simulink model "Control_model_matching_no_lineal"  (R2023a)
settings: Solver=FixedStepAuto  StartTime=0.0  StopTime=70  FixedStep=Ts  RelTol=1e-3
values from neighbouring files (symbols this model uses):
  IMU1_aB = [0.000820278190076 0.00115353439469 0.000894968456123]    [DatosSimulador.mat]
  IMU1_aK = [1.26449540403e-05 4.27040286013e-05 5.33261409146e-05]    [DatosSimulador.mat]
  IMU1_aN = [0.00684624677524 0.00597589835525 0.00590605800971]    [DatosSimulador.mat]
  IMU1_gB = [0.000430438056355 0.000168108439539 0.000519584631547]    [DatosSimulador.mat]
  IMU1_gK = [3.54504736606e-05 3.3319713566e-06 4.94506384712e-05]    [DatosSimulador.mat]
  IMU1_gN = [0.0047084921971 0.00506619736552 0.00340488785878]    [DatosSimulador.mat]
  IMU2_aB = [0.00173700635787 0.00079356651986 0.000918277248275]    [DatosSimulador.mat]
  IMU2_aK = [0.000253509817412 2.45614519372e-05 6.68535212753e-05]    [DatosSimulador.mat]
  IMU2_aN = [0.00535466242582 0.00533867441118 0.00558323645964]    [DatosSimulador.mat]
  IMU2_gB = [0.000335599994287 0.000795064377598 0.00045980210416]    [DatosSimulador.mat]
  IMU2_gK = [3.18091115332e-05 5.54514226678e-05 3.22930100083e-05]    [DatosSimulador.mat]
  IMU2_gN = [0.00695891398937 0.00398353487253 0.00368572026491]    [DatosSimulador.mat]
  IMU3_aB = [0.000325683271512 0.000441587151727 0.000601047067903]    [DatosSimulador.mat]
  IMU3_aK = [1.00979314084e-05 2.18555360334e-05 3.5534689232e-05]    [DatosSimulador.mat]
  IMU3_aN = [0.00413628574461 0.00448110466823 0.00368606415577]    [DatosSimulador.mat]
  IMU3_gB = [0.000501559406985 0.000889874761924 0.000218087094254]    [DatosSimulador.mat]
  IMU3_gK = [1.959913061e-05 4.03655103582e-05 4.44406532552e-06]    [DatosSimulador.mat]
  IMU3_gN = [0.00573350535706 0.0096154846251 0.00568739091977]    [DatosSimulador.mat]
  Ts = 0.001    [DatosSimulador.mat]
  TsMot = 0.001    [DatosSimulador.mat]
  TsPos = 0.002    [DatosSimulador.mat]
  TsRef = 0.02    [DatosSimulador.mat]
  TsSenB = 0.001    [DatosSimulador.mat]
  TsSenF = 0.001    [DatosSimulador.mat]
  TsVel = 0.001    [DatosSimulador.mat]
undefined symbols (not defined in the file or in its folder): denG, denM, numG, numM
libraries: mspsensorlib x3, simulink x2
(part 2 of 3)

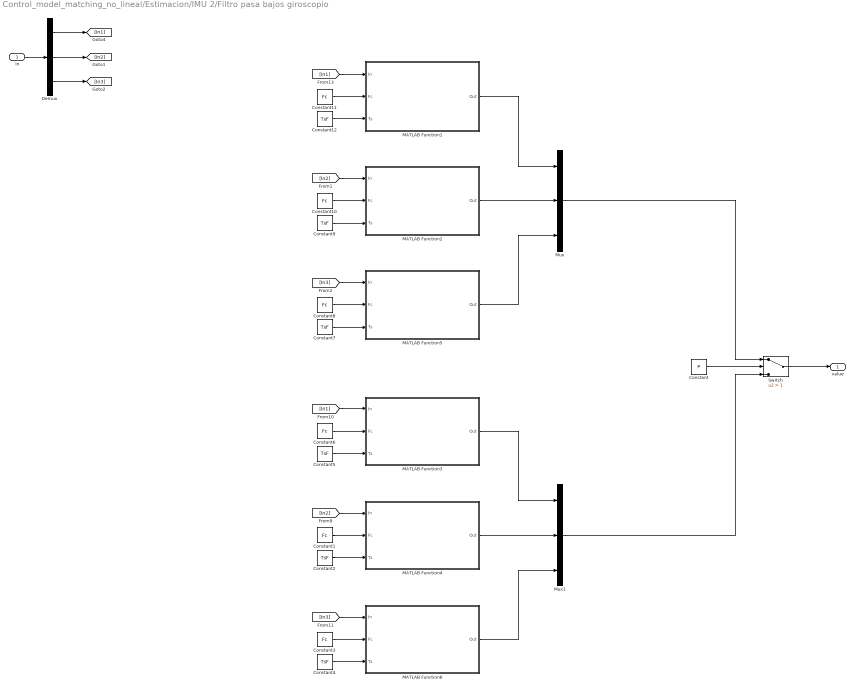
== system Control_model_matching_no_lineal/Estimacion/IMU 2/Filtro pasa bajos giroscopio ==
  In : Inport
  Constant : Constant  Value=P
  Constant{1,3,6,8,10..11} (6 alike) : Constant  Value=Fc
  Constant{2,4..5,7,9,12} (6 alike) : Constant  Value=TsF
  Demux : Demux  Outputs=3
  MATLAB Function1 : MATLAB Function  TreatAsAtomicUnit=on
  MATLAB Function2 : MATLAB Function  TreatAsAtomicUnit=on
  MATLAB Function3 : MATLAB Function  TreatAsAtomicUnit=on
  MATLAB Function4 : MATLAB Function  TreatAsAtomicUnit=on
  MATLAB Function5 : MATLAB Function  TreatAsAtomicUnit=on
  MATLAB Function6 : MATLAB Function  TreatAsAtomicUnit=on
  Mux : Mux  Inputs=3
  Mux1 : Mux  Inputs=3
  Switch : Switch  Criteria=u2 > Threshold  Threshold=1  SaturateOnIntegerOverflow=off  InputSameDT=off
  value : Outport
  wires:
  Constant/1 -> Switch/2
  Switch/1 -> value/1
  [In1] -> MATLAB Function1/1(In)
  MATLAB Function2/1(Out) -> Mux/2
  MATLAB Function1/1(Out) -> Mux/1
  MATLAB Function5/1(Out) -> Mux/3
  Mux/1 -> Switch/1
  In/1 -> Demux/1
  Demux/1 -> [In1]
  Demux/2 -> [In2]
  Demux/3 -> [In3]
  [In2] -> MATLAB Function2/1(In)
  [In3] -> MATLAB Function5/1(In)
  Constant4/1 -> MATLAB Function6/3(Ts)
  Constant3/1 -> MATLAB Function6/2(Fc)
  Constant1/1 -> MATLAB Function4/2(Fc)
  Constant2/1 -> MATLAB Function4/3(Ts)
  [In3] -> MATLAB Function6/1(In)
  [In2] -> MATLAB Function4/1(In)
  [In1] -> MATLAB Function3/1(In)
  MATLAB Function3/1(Out) -> Mux1/1
  MATLAB Function4/1(Out) -> Mux1/2
  MATLAB Function6/1(Out) -> Mux1/3
  Mux1/1 -> Switch/3
  Constant5/1 -> MATLAB Function3/3(Ts)
  Constant6/1 -> MATLAB Function3/2(Fc)
  Constant7/1 -> MATLAB Function5/3(Ts)
  Constant8/1 -> MATLAB Function5/2(Fc)
  Constant10/1 -> MATLAB Function2/2(Fc)
  Constant9/1 -> MATLAB Function2/3(Ts)
  Constant12/1 -> MATLAB Function1/3(Ts)
  Constant11/1 -> MATLAB Function1/2(Fc)

== system Control_model_matching_no_lineal/Estimacion/IMU 2/Sensor IMU ==
  GirT : Inport
  AcelT : Inport  Port=2
  Q : Inport  Port=3
  Constant : Constant  Value=R
  Constant1 : Constant  Value=R
  Gain1 : Gain  Gain=pi/180
  Gain3 : Gain  Gain=180/pi
  Gain4 : Gain  Gain=1/9.81
  IMU : mspsensorlib/IMU  DispRefFrame=NED  Temperature=25  MagneticFieldNED=[ 27.5550, -2.4169, -16.0849 ]  MagneticFieldENU=[ -2.4169, 27.5550, 16.0849 ]  SeedDouble=67  SimulateUsing=Code generation  AccelParamsMeasurementRange=156.9048  AccelParamsResolution=0  AccelParamsConstantBias=[0.0 0.0 0.0]  AccelParamsAxesMisalignment=[0 0 0]  AccelParamsNoiseDensity=aN  AccelParamsBiasInstability=aB  AccelParamsRandomWalk=aK  AccelParamsTemperatureBias=[0 0 0]  AccelParamsTemperatureScaleFactor=[0 0 0]  GyroParamsMeasurementRange=34.9066  GyroParamsResolution=0  GyroParamsConstantBias=[0.0 0.0 0.0]  GyroParamsAxesMisalignment=0  GyroParamsAccelerationBias=[0 0 0]  GyroParamsNoiseDensity=gN  GyroParamsBiasInstability=gB  GyroParamsRandomWalk=gK  GyroParamsTemperatureBias=[0 0 0]  GyroParamsTemperatureScaleFactor=[0 0 0]  MagParamsMeasurementRange=1000  MagParamsResolution=0.1  MagParamsConstantBias=0  MagParamsAxesMisalignment=[0 0 0]  MagParamsNoiseDensity=[0.0424 0.0424 0.0424]  MagParamsBiasInstability=[0 0 0]  MagParamsRandomWalk=[0 0 0]  MagParamsTemperatureBias=[0 0 0]  MagParamsTemperatureScaleFactor=[0 0 0]
  MATLAB Function5 : MATLAB Function  TreatAsAtomicUnit=on  SystemSampleTime=Ts
  Mux : Mux  Inputs=3
  Mux1 : Mux  Inputs=3
  Random Number : RandomNumber  Variance=0.1492^2*1000  SampleTime=Ts
  Random Number3 : RandomNumber  Variance=0.0154^2*1000  SampleTime=Ts
  Sum : Sum  Inputs=|++
  Sum1 : Sum  Inputs=|++
  Switch1 : Switch  Criteria=u2 > Threshold  SaturateOnIntegerOverflow=off  InputSameDT=off
  Switch2 : Switch  Criteria=u2 > Threshold  SaturateOnIntegerOverflow=off  InputSameDT=off
  Transpose1 : Math  Operator=transpose
  Transpose2 : Math  Operator=transpose
  Transpose3 : Math  Operator=transpose
  Zero-Order Hold : ZeroOrderHold  SampleTime=Ts
  Zero-Order Hold1 : ZeroOrderHold  SampleTime=Ts
  Zero-Order Hold2 : ZeroOrderHold  SampleTime=Ts
  AcelB : Outport
  VelB : Outport  Port=2
  wires:
  Zero-Order Hold2/1 -> MATLAB Function5/2(Q), IMU/3
  Zero-Order Hold1/1 -> MATLAB Function5/1(Wb)
  Zero-Order Hold/1 -> Transpose2/1
  Switch1/1 -> IMU/2
  Switch2/1 -> IMU/1
  Gain1/1 -> Sum1/2, Switch1/3
  Sum1/1 -> Switch1/1
  Constant1/1 -> Switch1/2
  Constant/1 -> Switch2/2
  Sum/1 -> Switch2/1
  Random Number3/1 -> Mux1/3, Mux1/2, Mux1/1
  Mux1/1 -> Sum1/1
  Transpose2/1 -> Sum/2, Switch2/3
  Mux/1 -> Sum/1
  Random Number/1 -> Mux/1, Mux/3, Mux/2
  Q/1 -> Zero-Order Hold2/1
  MATLAB Function5/1(Vel) -> Gain1/1
  Transpose3/1 -> Gain3/1
  IMU/1 -> Transpose1/1
  IMU/2 -> Transpose3/1
  GirT/1 -> Zero-Order Hold1/1
  AcelT/1 -> Zero-Order Hold/1
  Transpose1/1 -> Gain4/1
  Gain4/1 -> AcelB/1
  Gain3/1 -> VelB/1

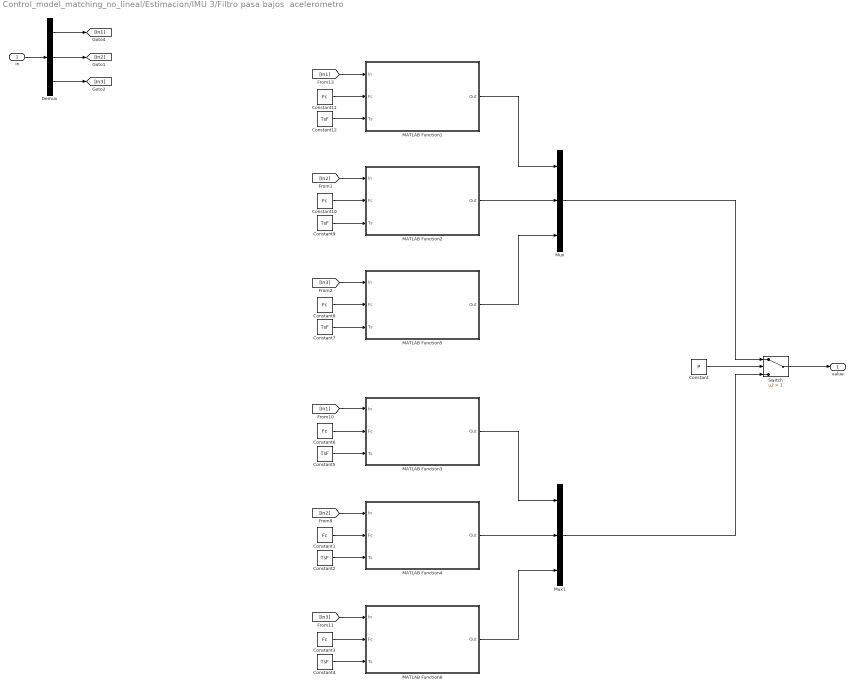
== system Control_model_matching_no_lineal/Estimacion/IMU 3/Filtro pasa bajos  acelerometro ==
  In : Inport
  Constant : Constant  Value=P
  Constant{1,3,6,8,10..11} (6 alike) : Constant  Value=Fc
  Constant{2,4..5,7,9,12} (6 alike) : Constant  Value=TsF
  Demux : Demux  Outputs=3
  MATLAB Function1 : MATLAB Function  TreatAsAtomicUnit=on
  MATLAB Function2 : MATLAB Function  TreatAsAtomicUnit=on
  MATLAB Function3 : MATLAB Function  TreatAsAtomicUnit=on
  MATLAB Function4 : MATLAB Function  TreatAsAtomicUnit=on
  MATLAB Function5 : MATLAB Function  TreatAsAtomicUnit=on
  MATLAB Function6 : MATLAB Function  TreatAsAtomicUnit=on
  Mux : Mux  Inputs=3
  Mux1 : Mux  Inputs=3
  Switch : Switch  Criteria=u2 > Threshold  Threshold=1  SaturateOnIntegerOverflow=off  InputSameDT=off
  value : Outport
  wires:
  Constant/1 -> Switch/2
  Switch/1 -> value/1
  [In1] -> MATLAB Function1/1(In)
  MATLAB Function2/1(Out) -> Mux/2
  MATLAB Function1/1(Out) -> Mux/1
  MATLAB Function5/1(Out) -> Mux/3
  Mux/1 -> Switch/1
  In/1 -> Demux/1
  Demux/1 -> [In1]
  Demux/2 -> [In2]
  Demux/3 -> [In3]
  [In2] -> MATLAB Function2/1(In)
  [In3] -> MATLAB Function5/1(In)
  Constant4/1 -> MATLAB Function6/3(Ts)
  Constant3/1 -> MATLAB Function6/2(Fc)
  Constant1/1 -> MATLAB Function4/2(Fc)
  Constant2/1 -> MATLAB Function4/3(Ts)
  [In3] -> MATLAB Function6/1(In)
  [In2] -> MATLAB Function4/1(In)
  [In1] -> MATLAB Function3/1(In)
  MATLAB Function3/1(Out) -> Mux1/1
  MATLAB Function4/1(Out) -> Mux1/2
  MATLAB Function6/1(Out) -> Mux1/3
  Mux1/1 -> Switch/3
  Constant5/1 -> MATLAB Function3/3(Ts)
  Constant6/1 -> MATLAB Function3/2(Fc)
  Constant7/1 -> MATLAB Function5/3(Ts)
  Constant8/1 -> MATLAB Function5/2(Fc)
  Constant10/1 -> MATLAB Function2/2(Fc)
  Constant9/1 -> MATLAB Function2/3(Ts)
  Constant12/1 -> MATLAB Function1/3(Ts)
  Constant11/1 -> MATLAB Function1/2(Fc)

== system Control_model_matching_no_lineal/Estimacion/IMU 3/Filtro pasa bajos giroscopio ==
  In : Inport
  Constant : Constant  Value=P
  Constant{1,3,6,8,10..11} (6 alike) : Constant  Value=Fc
  Constant{2,4..5,7,9,12} (6 alike) : Constant  Value=TsF
  Demux : Demux  Outputs=3
  MATLAB Function1 : MATLAB Function  TreatAsAtomicUnit=on
  MATLAB Function2 : MATLAB Function  TreatAsAtomicUnit=on
  MATLAB Function3 : MATLAB Function  TreatAsAtomicUnit=on
  MATLAB Function4 : MATLAB Function  TreatAsAtomicUnit=on
  MATLAB Function5 : MATLAB Function  TreatAsAtomicUnit=on
  MATLAB Function6 : MATLAB Function  TreatAsAtomicUnit=on
  Mux : Mux  Inputs=3
  Mux1 : Mux  Inputs=3
  Switch : Switch  Criteria=u2 > Threshold  Threshold=1  SaturateOnIntegerOverflow=off  InputSameDT=off
  value : Outport
  wires:
  Constant11/1 -> MATLAB Function1/2(Fc)
  Constant12/1 -> MATLAB Function1/3(Ts)
  Constant9/1 -> MATLAB Function2/3(Ts)
  Constant10/1 -> MATLAB Function2/2(Fc)
  Constant8/1 -> MATLAB Function5/2(Fc)
  Constant7/1 -> MATLAB Function5/3(Ts)
  Constant6/1 -> MATLAB Function3/2(Fc)
  Constant5/1 -> MATLAB Function3/3(Ts)
  Mux1/1 -> Switch/3
  MATLAB Function6/1(Out) -> Mux1/3
  MATLAB Function4/1(Out) -> Mux1/2
  MATLAB Function3/1(Out) -> Mux1/1
  [In1] -> MATLAB Function3/1(In)
  [In2] -> MATLAB Function4/1(In)
  [In3] -> MATLAB Function6/1(In)
  Constant2/1 -> MATLAB Function4/3(Ts)
  Constant1/1 -> MATLAB Function4/2(Fc)
  Constant3/1 -> MATLAB Function6/2(Fc)
  Constant4/1 -> MATLAB Function6/3(Ts)
  [In3] -> MATLAB Function5/1(In)
  [In2] -> MATLAB Function2/1(In)
  Demux/3 -> [In3]
  Demux/2 -> [In2]
  Demux/1 -> [In1]
  In/1 -> Demux/1
  Mux/1 -> Switch/1
  MATLAB Function5/1(Out) -> Mux/3
  MATLAB Function1/1(Out) -> Mux/1
  MATLAB Function2/1(Out) -> Mux/2
  [In1] -> MATLAB Function1/1(In)
  Switch/1 -> value/1
  Constant/1 -> Switch/2

== system Control_model_matching_no_lineal/Estimacion/IMU 3/Sensor IMU ==
  GirT : Inport
  AcelT : Inport  Port=2
  Q : Inport  Port=3
  Constant : Constant  Value=R
  Constant1 : Constant  Value=R
  Gain1 : Gain  Gain=pi/180
  Gain3 : Gain  Gain=180/pi
  Gain4 : Gain  Gain=1/9.81
  IMU : mspsensorlib/IMU  DispRefFrame=NED  Temperature=25  MagneticFieldNED=[ 27.5550, -2.4169, -16.0849 ]  MagneticFieldENU=[ -2.4169, 27.5550, 16.0849 ]  SeedDouble=67  SimulateUsing=Code generation  AccelParamsMeasurementRange=156.9048  AccelParamsResolution=0  AccelParamsConstantBias=[0.0 0.0 0.0]  AccelParamsAxesMisalignment=[0 0 0]  AccelParamsNoiseDensity=aN  AccelParamsBiasInstability=aB  AccelParamsRandomWalk=aK  AccelParamsTemperatureBias=[0 0 0]  AccelParamsTemperatureScaleFactor=[0 0 0]  GyroParamsMeasurementRange=34.9066  GyroParamsResolution=0  GyroParamsConstantBias=[0.0 0.0 0.0]  GyroParamsAxesMisalignment=0  GyroParamsAccelerationBias=[0 0 0]  GyroParamsNoiseDensity=gN  GyroParamsBiasInstability=gB  GyroParamsRandomWalk=gK  GyroParamsTemperatureBias=[0 0 0]  GyroParamsTemperatureScaleFactor=[0 0 0]  MagParamsMeasurementRange=1000  MagParamsResolution=0.1  MagParamsConstantBias=0  MagParamsAxesMisalignment=[0 0 0]  MagParamsNoiseDensity=[0.0424 0.0424 0.0424]  MagParamsBiasInstability=[0 0 0]  MagParamsRandomWalk=[0 0 0]  MagParamsTemperatureBias=[0 0 0]  MagParamsTemperatureScaleFactor=[0 0 0]
  MATLAB Function5 : MATLAB Function  TreatAsAtomicUnit=on  SystemSampleTime=Ts
  Mux : Mux  Inputs=3
  Mux1 : Mux  Inputs=3
  Random Number : RandomNumber  Variance=0.1492^2*1000  SampleTime=Ts
  Random Number3 : RandomNumber  Variance=0.0154^2*1000  SampleTime=Ts
  Sum : Sum  Inputs=|++
  Sum1 : Sum  Inputs=|++
  Switch1 : Switch  Criteria=u2 > Threshold  SaturateOnIntegerOverflow=off  InputSameDT=off
  Switch2 : Switch  Criteria=u2 > Threshold  SaturateOnIntegerOverflow=off  InputSameDT=off
  Transpose1 : Math  Operator=transpose
  Transpose2 : Math  Operator=transpose
  Transpose3 : Math  Operator=transpose
  Zero-Order Hold : ZeroOrderHold  SampleTime=Ts
  Zero-Order Hold1 : ZeroOrderHold  SampleTime=Ts
  Zero-Order Hold2 : ZeroOrderHold  SampleTime=Ts
  AcelB : Outport
  VelB : Outport  Port=2
  wires:
  Gain3/1 -> VelB/1
  Gain4/1 -> AcelB/1
  Transpose1/1 -> Gain4/1
  AcelT/1 -> Zero-Order Hold/1
  GirT/1 -> Zero-Order Hold1/1
  IMU/2 -> Transpose3/1
  IMU/1 -> Transpose1/1
  Transpose3/1 -> Gain3/1
  MATLAB Function5/1(Vel) -> Gain1/1
  Q/1 -> Zero-Order Hold2/1
  Random Number/1 -> Mux/2, Mux/3, Mux/1
  Mux/1 -> Sum/1
  Transpose2/1 -> Switch2/3, Sum/2
  Mux1/1 -> Sum1/1
  Random Number3/1 -> Mux1/1, Mux1/2, Mux1/3
  Sum/1 -> Switch2/1
  Constant/1 -> Switch2/2
  Constant1/1 -> Switch1/2
  Sum1/1 -> Switch1/1
  Gain1/1 -> Switch1/3, Sum1/2
  Switch2/1 -> IMU/1
  Switch1/1 -> IMU/2
  Zero-Order Hold/1 -> Transpose2/1
  Zero-Order Hold1/1 -> MATLAB Function5/1(Wb)
  Zero-Order Hold2/1 -> IMU/3, MATLAB Function5/2(Q)

== matlab function Control_model_matching_no_lineal/Modelo UAV/Sistema de propulsion/MATLAB Function2 ==
  data: u input; v input; y output; vMin input; vMax input; m input
function y = fuerzaMotor(u, v, vMin, vMax, m)

f  = [0.0 0.0 0.0 0.0];
y1 = [0.0 0.0 0.0 0.0];
y2 = [0.0 0.0 0.0 0.0];
    
if v < vMin 
    t = vMin;
elseif v > vMax
    t = vMax;
else
    t = v;
end

nDim   = size(m, 1);
paso   = (vMax - vMin) / (nDim - 1);
nPasos = fix((t - vMin) / paso);
v1     = vMin + nPasos * paso;

% Filas de la matriz
x1 = nPasos + 1;
x2 = x1 + 1;


% Calculo de los puntos
for i = 1 : 4
    y1(i) = m(x1,1) * u(i)^3 + m(x1,2) * u(i)^2 + m(x1,3) * u(i) + m(x1,4); 
    y2(i) = m(x2,1) * u(i)^3 + m(x2,2) * u(i)^2 + m(x2,3) * u(i) + m(x2,4);

    % Interpolacion
    f(i) = y1(i) + (y2(i) - y1(i)) / paso * (t - v1);
end

y = f;

== matlab function Control_model_matching_no_lineal/Modelo UAV/Sistema de propulsion/MATLAB Function1 ==
  data: u input; v input; y output; vMin input; vMax input; m input
function y = dragMotor(u, v, vMin, vMax, m)

f  = [0.0 0.0 0.0 0.0];
y1 = [0.0 0.0 0.0 0.0];
y2 = [0.0 0.0 0.0 0.0];
    
if v < vMin 
    t = vMin;
elseif v > vMax
    t = vMax;
else
    t = v;
end

nDim   = size(m, 1);
paso   = (vMax - vMin) / (nDim - 1);
nPasos = fix((t - vMin) / paso);
v1     = vMin + nPasos * paso;

% Filas de la matriz
x1 = nPasos + 1;
x2 = x1 + 1;


% Calculo de los puntos
for i = 1 : 4
    y1(i) = m(x1,1) * u(i)^3 + m(x1,2) * u(i)^2 + m(x1,3) * u(i) + m(x1,4); 
    y2(i) = m(x2,1) * u(i)^3 + m(x2,2) * u(i)^2 + m(x2,3) * u(i) + m(x2,4);

    % Interpolacion
    f(i) = y1(i) + (y2(i) - y1(i)) / paso * (t - v1);
end

y = f;

== matlab function Control_model_matching_no_lineal/Modelo UAV/Sistema de propulsion/MATLAB Function3 ==
  data: u input; v input; y output; vMin input; vMax input; m input
function y = velMotor(u, v, vMin, vMax, m)

f  = [0.0 0.0 0.0 0.0];
y1 = [0.0 0.0 0.0 0.0];
y2 = [0.0 0.0 0.0 0.0];
    
if v < vMin 
    t = vMin;
elseif v > vMax
    t = vMax;
else
    t = v;
end

nDim   = size(m, 1);
paso   = (vMax - vMin) / (nDim - 1);
nPasos = fix((t - vMin) / paso);
v1     = vMin + nPasos * paso;

% Filas de la matriz
x1 = nPasos + 1;
x2 = x1 + 1;


% Calculo de los puntos
for i = 1 : 4
    y1(i) = m(x1,1) * u(i)^3 + m(x1,2) * u(i)^2 + m(x1,3) * u(i) + m(x1,4); 
    y2(i) = m(x2,1) * u(i)^3 + m(x2,2) * u(i)^2 + m(x2,3) * u(i) + m(x2,4);

    % Interpolacion
    f(i) = y1(i) + (y2(i) - y1(i)) / paso * (t - v1);
end

y = f;

== matlab function Control_model_matching_no_lineal/Estimacion/AHRS/MATLAB Function2 ==
  data: kp input; ki input; gir input; acel input; tiempo input; Q output
function Q = Mahony(kp, ki, gir, acel, tiempo)

persistent tiempoAnterior q ei

if isempty(tiempoAnterior)
    tiempoAnterior = 0;
    q  = [1 0 0 0]';
    ei = [0 0 0]';
end

v   = [0 0 0]';
e   = [0 0 0]';
vel = [0 0 0]';

dt = tiempo - tiempoAnterior;
tiempoAnterior = tiempo;

if (~((acel(1) == 0) && (acel(2) == 0) && (acel(3) == 0))) 

	% Se normaliza la acelereacion
    normA = norm(acel);
    if normA ~= 0 
        a = acel / normA;
    else
        a = acel;
    end

    % Direccion estimada de la gravedad
    v(1) = q(2) * q(4) - q(1) * q(3);
    v(2) = q(1) * q(2) + q(3) * q(4);
    v(3) = q(1) * q(1) - 0.5 + q(4) * q(4);

    % El error es la suma del producto cruzado entre la dirección de gravedad estimada y medida
    e(1) = (a(2) * v(3) - a(3) * v(2));
    e(2) = (a(3) * v(1) - a(1) * v(3));
    e(3) = (a(1) * v(2) - a(2) * v(1));

    vel = gir;

	% Calcular y aplica el feedback integral si esta habilitado
    if ki > 0.0
        ei(1) = ei(1) + ki * e(1) * dt;
        ei(2) = ei(2) + ki * e(2) * dt;
        ei(3) = ei(3) + ki * e(3) * dt;

        vel(1) = vel(1) + ei(1);
        vel(2) = vel(2) + ei(2);
        vel(3) = vel(3) + ei(3);
    else 
		ei(1) = 0.0;	% Anti wind-up
		ei(2) = 0.0;
		ei(3) = 0.0;
    end

    % Ganancia proporcional
    vel(1) = vel(1) + kp * e(1);
    vel(2) = vel(2) + kp * e(2);
    vel(3) = vel(3) + kp * e(3);
end

% Se integra la tasa de cambio de cuaternion
vel(1) = vel(1) * (0.5 * dt);
vel(2) = vel(2) * (0.5 * dt);
vel(3) = vel(3) * (0.5 * dt);

q1 = q(1);
q2 = q(2);
q3 = q(3);

q(1) = q(1) + (-q2 * vel(1) - q3 * vel(2) - q(4) * vel(3));
q(2) = q(2) + ( q1 * vel(1) + q3 * vel(3) - q(4) * vel(2));
q(3) = q(3) + ( q1 * vel(2) - q2 * vel(3) + q(4) * vel(1));
q(4) = q(4) + ( q1 * vel(3) + q2 * vel(2) - q3   * vel(1));


% Se normaliza el cuaternion
Q = q / norm(q);

== matlab function Control_model_matching_no_lineal/Estimacion/MATLAB Function1 ==
  data: acel input; acelV output; gir input; girV output
function [acelV, girV] = ImuVirtual(acel, gir)

acelAcum = [0 0 0]';
girAcum  = [0 0 0]';

for ind = 1 : 3
    i = (ind - 1) * 3 + 1;

    acelAcum(1) = acelAcum(1) + acel(i);
    acelAcum(2) = acelAcum(2) + acel(i+1);
    acelAcum(3) = acelAcum(3) + acel(i+2);

    girAcum(1) = girAcum(1) + gir(i);
    girAcum(2) = girAcum(2) + gir(i+1);
    girAcum(3) = girAcum(3) + gir(i+2);
end

acelV = acelAcum / 3;
girV  = girAcum  / 3;

== matlab function Control_model_matching_no_lineal/Sistema de control/MATLAB Function ==
  data: u input; pwm output size=4
function pwm = Mixer(u)
    pwm = [0 0 0 0]';
    
    pwm(1) = u(4) - u(1) + u(2) + u(3);
    pwm(2) = u(4) + u(1) + u(2) - u(3);
    pwm(3) = u(4) + u(1) - u(2) + u(3);   
    pwm(4) = u(4) - u(1) - u(2) - u(3);

== matlab function Control_model_matching_no_lineal/Modelo UAV/Dinamica UAV/Rotacion ==
  settings: updateMethod=DISCRETE
  data: Q output; Wb input size=3; Euler output size=3; Tiempo input
function [Q, Euler] = RotacionAngular(Wb, Tiempo)

persistent q TiempoAnterior

if isempty(q)
    q  = [1 0 0 0];
    TiempoAnterior = 0;
end

dt = Tiempo - TiempoAnterior;
TiempoAnterior = Tiempo;

W = [0 0 0]';
Euler = [0 0 0]';

% Se integra la tasa de cambio de cuaternion
W(1) = Wb(1) * (0.5 * dt);
W(2) = Wb(2) * (0.5 * dt);
W(3) = Wb(3) * (0.5 * dt);

q1 = q(1);
q2 = q(2);
q3 = q(3);

q(1) = q(1) + (-q2 * W(1) - q3 * W(2) - q(4) * W(3));
q(2) = q(2) + ( q1 * W(1) + q3 * W(3) - q(4) * W(2));
q(3) = q(3) + ( q1 * W(2) - q2 * W(3) + q(4) * W(1));
q(4) = q(4) + ( q1 * W(3) + q2 * W(2) - q3   * W(1));


% Se normaliza el cuaternion
Q = q / norm(q);

% Ecuaciones sacadas de Madgwick con el conjugado implicito en las formulas
Euler(1) = atan2(2 * Q(3) * Q(4) + 2 * Q(1) * Q(2), 2 * Q(1) * Q(1) + 2 * Q(4) * Q(4) - 1);
Euler(2) = -asin(2 * (Q(2) * Q(4) - Q(1) * Q(3)));
Euler(3) = atan2(2 * Q(2) * Q(3) + 2 * Q(1) * Q(4), 2 * Q(1) * Q(1) + 2 * Q(2) * Q(2) - 1);

== matlab function Control_model_matching_no_lineal/Estimacion/AHRS/MATLAB Function4 ==
  data: Q input; Euler output
function Euler = AHRS(Q)

euler = [0 0 0];

% Ecuaciones sacadas de Madgwick con el conjugado implicito en las formulas
euler(1) = atan2(2 * Q(3) * Q(4) + 2 * Q(1) * Q(2), 2 * Q(1) * Q(1) + 2 * Q(4) * Q(4) - 1);
euler(2) = -asin(2 * (Q(2) * Q(4) - Q(1) * Q(3)));
euler(3) = atan2(2 * Q(2) * Q(3) + 2 * Q(1) * Q(4), 2 * Q(1) * Q(1) + 2 * Q(2) * Q(2) - 1);

% Conversion a grados
euler = euler * 180 / pi;

% Se convierte el angulo de -180 a 180 a 0 360
if (euler(3) < 0)
	euler(3) = euler(3) + 360;
end

Euler = euler;

== matlab function Control_model_matching_no_lineal/Estimacion/IMU 1/Filtro pasa bajos  acelerometro/MATLAB Function1 ==
  settings: updateMethod=DISCRETE
  data: In input; Fc input; Out output; Ts input
function Out  = LowPassFilterP2(In, Fc, Ts)

persistent b0 b1 b2 a1 a2 a0 in1 in2 out1 out2

if isempty(b0)
    ohm     = 2 * pi * Fc;
    damping = 1 / (sqrt(2));

    b2 = Ts^2 * ohm^2;
    b1 = 2.0 * b2;
    b0 = b2;

    a2 = 4.0 + 4.0 * damping * ohm * Ts + b2;
    a1 = -8.0 + b1;
    a0 = 4.0 - 4.0 * damping * ohm * Ts + b2;

    in1  = 0;
    in2  = 0;
    out1 = 0;
    out2 = 0;
end

Out = (b2 * In + b1 * in1 + b0 * in2 - a1 * out1 - a0 * out2) / a2;

in2  = in1;
in1  = In;
out2 = out1;
out1 = Out;

== matlab function Control_model_matching_no_lineal/Estimacion/IMU 2/Filtro pasa bajos  acelerometro/MATLAB Function1 ==
  settings: updateMethod=DISCRETE
  data: In input; Fc input; Out output; Ts input
function Out  = LowPassFilterP2(In, Fc, Ts)

persistent b0 b1 b2 a1 a2 a0 in1 in2 out1 out2

if isempty(b0)
    ohm     = 2 * pi * Fc;
    damping = 1 / (sqrt(2));

    b2 = Ts^2 * ohm^2;
    b1 = 2.0 * b2;
    b0 = b2;

    a2 = 4.0 + 4.0 * damping * ohm * Ts + b2;
    a1 = -8.0 + b1;
    a0 = 4.0 - 4.0 * damping * ohm * Ts + b2;

    in1  = 0;
    in2  = 0;
    out1 = 0;
    out2 = 0;
end

Out = (b2 * In + b1 * in1 + b0 * in2 - a1 * out1 - a0 * out2) / a2;

in2  = in1;
in1  = In;
out2 = out1;
out1 = Out;

== matlab function Control_model_matching_no_lineal/Estimacion/IMU 2/Filtro pasa bajos  acelerometro/MATLAB Function2 ==
  settings: updateMethod=DISCRETE
  data: In input; Fc input; Out output; Ts input
function Out  = LowPassFilterP2(In, Fc, Ts)

persistent b0 b1 b2 a1 a2 a0 in1 in2 out1 out2

if isempty(b0)
    ohm     = 2 * pi * Fc;
    damping = 1 / (sqrt(2));

    b2 = Ts^2 * ohm^2;
    b1 = 2.0 * b2;
    b0 = b2;

    a2 = 4.0 + 4.0 * damping * ohm * Ts + b2;
    a1 = -8.0 + b1;
    a0 = 4.0 - 4.0 * damping * ohm * Ts + b2;

    in1  = 0;
    in2  = 0;
    out1 = 0;
    out2 = 0;
end

Out = (b2 * In + b1 * in1 + b0 * in2 - a1 * out1 - a0 * out2) / a2;

in2  = in1;
in1  = In;
out2 = out1;
out1 = Out;

== matlab function Control_model_matching_no_lineal/Estimacion/IMU 2/Filtro pasa bajos  acelerometro/MATLAB Function3 ==
  settings: updateMethod=DISCRETE
  data: In input; Fc input; Out output; Ts input
function Out  = LowPassFilterP1(In, Fc, Ts)

persistent b0 b1 a0 a1 in1 out1

if isempty(b0)
    ohm = 2.0 * pi * Fc;

    b1 = ohm * Ts;
    b0 = b1;
    a1 = 2.0 + b1;
    a0 = b1 - 2.0;

    in1  = 0;
    out1 = 0;
end

Out = (b1 * In + b0 * in1 - a0 * out1) / a1;

in1  = In;
out1 = Out;

== matlab function Control_model_matching_no_lineal/Estimacion/IMU 2/Filtro pasa bajos  acelerometro/MATLAB Function4 ==
  settings: updateMethod=DISCRETE
  data: In input; Fc input; Out output; Ts input
function Out  = LowPassFilterP1(In, Fc, Ts)

persistent b0 b1 a0 a1 in1 out1

if isempty(b0)
    ohm = 2.0 * pi * Fc;

    b1 = ohm * Ts;
    b0 = b1;
    a1 = 2.0 + b1;
    a0 = b1 - 2.0;

    in1  = 0;
    out1 = 0;
end

Out = (b1 * In + b0 * in1 - a0 * out1) / a1;

in1  = In;
out1 = Out;

== matlab function Control_model_matching_no_lineal/Estimacion/IMU 2/Filtro pasa bajos  acelerometro/MATLAB Function5 ==
  settings: updateMethod=DISCRETE
  data: In input; Fc input; Out output; Ts input
function Out  = LowPassFilterP2(In, Fc, Ts)

persistent b0 b1 b2 a1 a2 a0 in1 in2 out1 out2

if isempty(b0)
    ohm     = 2 * pi * Fc;
    damping = 1 / (sqrt(2));

    b2 = Ts^2 * ohm^2;
    b1 = 2.0 * b2;
    b0 = b2;

    a2 = 4.0 + 4.0 * damping * ohm * Ts + b2;
    a1 = -8.0 + b1;
    a0 = 4.0 - 4.0 * damping * ohm * Ts + b2;

    in1  = 0;
    in2  = 0;
    out1 = 0;
    out2 = 0;
end

Out = (b2 * In + b1 * in1 + b0 * in2 - a1 * out1 - a0 * out2) / a2;

in2  = in1;
in1  = In;
out2 = out1;
out1 = Out;

== matlab function Control_model_matching_no_lineal/Estimacion/IMU 2/Filtro pasa bajos  acelerometro/MATLAB Function6 ==
  settings: updateMethod=DISCRETE
  data: In input; Fc input; Out output; Ts input
function Out  = LowPassFilterP1(In, Fc, Ts)

persistent b0 b1 a0 a1 in1 out1

if isempty(b0)
    ohm = 2.0 * pi * Fc;

    b1 = ohm * Ts;
    b0 = b1;
    a1 = 2.0 + b1;
    a0 = b1 - 2.0;

    in1  = 0;
    out1 = 0;
end

Out = (b1 * In + b0 * in1 - a0 * out1) / a1;

in1  = In;
out1 = Out;

== matlab function Control_model_matching_no_lineal/Estimacion/IMU 2/Filtro pasa bajos giroscopio/MATLAB Function1 ==
  settings: updateMethod=DISCRETE
  data: In input; Fc input; Out output; Ts input
function Out  = LowPassFilterP2(In, Fc, Ts)

persistent b0 b1 b2 a1 a2 a0 in1 in2 out1 out2

if isempty(b0)
    ohm     = 2 * pi * Fc;
    damping = 1 / (sqrt(2));

    b2 = Ts^2 * ohm^2;
    b1 = 2.0 * b2;
    b0 = b2;

    a2 = 4.0 + 4.0 * damping * ohm * Ts + b2;
    a1 = -8.0 + b1;
    a0 = 4.0 - 4.0 * damping * ohm * Ts + b2;

    in1  = 0;
    in2  = 0;
    out1 = 0;
    out2 = 0;
end

Out = (b2 * In + b1 * in1 + b0 * in2 - a1 * out1 - a0 * out2) / a2;

in2  = in1;
in1  = In;
out2 = out1;
out1 = Out;

== matlab function Control_model_matching_no_lineal/Estimacion/IMU 2/Filtro pasa bajos giroscopio/MATLAB Function2 ==
  settings: updateMethod=DISCRETE
  data: In input; Fc input; Out output; Ts input
function Out  = LowPassFilterP2(In, Fc, Ts)

persistent b0 b1 b2 a1 a2 a0 in1 in2 out1 out2

if isempty(b0)
    ohm     = 2 * pi * Fc;
    damping = 1 / (sqrt(2));

    b2 = Ts^2 * ohm^2;
    b1 = 2.0 * b2;
    b0 = b2;

    a2 = 4.0 + 4.0 * damping * ohm * Ts + b2;
    a1 = -8.0 + b1;
    a0 = 4.0 - 4.0 * damping * ohm * Ts + b2;

    in1  = 0;
    in2  = 0;
    out1 = 0;
    out2 = 0;
end

Out = (b2 * In + b1 * in1 + b0 * in2 - a1 * out1 - a0 * out2) / a2;

in2  = in1;
in1  = In;
out2 = out1;
out1 = Out;

== matlab function Control_model_matching_no_lineal/Estimacion/IMU 2/Filtro pasa bajos giroscopio/MATLAB Function3 ==
  settings: updateMethod=DISCRETE
  data: In input; Fc input; Out output; Ts input
function Out  = LowPassFilterP1(In, Fc, Ts)

persistent b0 b1 a0 a1 in1 out1

if isempty(b0)
    ohm = 2.0 * pi * Fc;

    b1 = ohm * Ts;
    b0 = b1;
    a1 = 2.0 + b1;
    a0 = b1 - 2.0;

    in1  = 0;
    out1 = 0;
end

Out = (b1 * In + b0 * in1 - a0 * out1) / a1;

in1  = In;
out1 = Out;

== matlab function Control_model_matching_no_lineal/Estimacion/IMU 2/Filtro pasa bajos giroscopio/MATLAB Function4 ==
  settings: updateMethod=DISCRETE
  data: In input; Fc input; Out output; Ts input
function Out  = LowPassFilterP1(In, Fc, Ts)

persistent b0 b1 a0 a1 in1 out1

if isempty(b0)
    ohm = 2.0 * pi * Fc;

    b1 = ohm * Ts;
    b0 = b1;
    a1 = 2.0 + b1;
    a0 = b1 - 2.0;

    in1  = 0;
    out1 = 0;
end

Out = (b1 * In + b0 * in1 - a0 * out1) / a1;

in1  = In;
out1 = Out;

== matlab function Control_model_matching_no_lineal/Estimacion/IMU 2/Filtro pasa bajos giroscopio/MATLAB Function5 ==
  settings: updateMethod=DISCRETE
  data: In input; Fc input; Out output; Ts input
function Out  = LowPassFilterP2(In, Fc, Ts)

persistent b0 b1 b2 a1 a2 a0 in1 in2 out1 out2

if isempty(b0)
    ohm     = 2 * pi * Fc;
    damping = 1 / (sqrt(2));

    b2 = Ts^2 * ohm^2;
    b1 = 2.0 * b2;
    b0 = b2;

    a2 = 4.0 + 4.0 * damping * ohm * Ts + b2;
    a1 = -8.0 + b1;
    a0 = 4.0 - 4.0 * damping * ohm * Ts + b2;

    in1  = 0;
    in2  = 0;
    out1 = 0;
    out2 = 0;
end

Out = (b2 * In + b1 * in1 + b0 * in2 - a1 * out1 - a0 * out2) / a2;

in2  = in1;
in1  = In;
out2 = out1;
out1 = Out;

== matlab function Control_model_matching_no_lineal/Estimacion/IMU 2/Filtro pasa bajos giroscopio/MATLAB Function6 ==
  settings: updateMethod=DISCRETE
  data: In input; Fc input; Out output; Ts input
function Out  = LowPassFilterP1(In, Fc, Ts)

persistent b0 b1 a0 a1 in1 out1

if isempty(b0)
    ohm = 2.0 * pi * Fc;

    b1 = ohm * Ts;
    b0 = b1;
    a1 = 2.0 + b1;
    a0 = b1 - 2.0;

    in1  = 0;
    out1 = 0;
end

Out = (b1 * In + b0 * in1 - a0 * out1) / a1;

in1  = In;
out1 = Out;

== matlab function Control_model_matching_no_lineal/Estimacion/IMU 2/MATLAB Function1 ==
  data: u input; max input; acumW2 data_store_memory; cntW2 data_store_memory
function escribirAcumuladorW(u, max)

global acumW2 cntW2

acumW2 = acumW2 + u;
cntW2  = cntW2 + 1;

if cntW2 >= max
    cntW2  = max / 2;
    acumW2 = acumW2 / 2;
end

== matlab function Control_model_matching_no_lineal/Estimacion/IMU 2/MATLAB Function2 ==
  data: y output; acumW2 data_store_memory; cntW2 data_store_memory
function y = leerAcumuladorW

global acumW2 cntW2
persistent valor

if isempty(valor)
    valor = [0 0 0]';
end

if cntW2 ~= 0
    valor  = acumW2 / cntW2;
    acumW2 = [0 0 0]';
    cntW2  = 0;
end
    
y = valor;

== matlab function Control_model_matching_no_lineal/Estimacion/IMU 2/MATLAB Function3 ==
  data: y output; acumA2 data_store_memory; cntA2 data_store_memory
function y = leerAcumuladorA

global acumA2 cntA2
persistent valor

if isempty(valor)
    valor = [0 0 0]';
end

if cntA2 ~= 0
    valor  = acumA2 / cntA2;
    acumA2 = [0 0 0]';
    cntA2  = 0;
end

y = valor;

== matlab function Control_model_matching_no_lineal/Estimacion/IMU 2/MATLAB Function4 ==
  data: u input; max input; acumA2 data_store_memory; cntA2 data_store_memory
function escribirAcumuladorA(u, max)

global acumA2 cntA2

acumA2 = acumA2 + u;
cntA2  = cntA2 + 1;

if cntA2 >= max
    cntA2 = max / 2;
    acumA2 = acumA2 / 2;
end

== matlab function Control_model_matching_no_lineal/Estimacion/IMU 2/Sensor IMU/MATLAB Function5 ==
  data: Wb input; Q input; Vel output
function Vel = RotacionVelBT(Wb, Q)

Euler = [0 0 0]';

Euler(1) = atan2(2 * Q(3) * Q(4) + 2 * Q(1) * Q(2), 2 * Q(1) * Q(1) + 2 * Q(4) * Q(4) - 1);
Euler(2) = -asin(2 * (Q(2) * Q(4) - Q(1) * Q(3)));
Euler(3) = atan2(2 * Q(2) * Q(3) + 2 * Q(1) * Q(4), 2 * Q(1) * Q(1) + 2 * Q(2) * Q(2) - 1);


w1 = Wb(1) + Wb(2) * sin(Euler(1)) * tan(Euler(2)) + Wb(3) * cos(Euler(1)) * tan(Euler(2));
w2 = Wb(2) * cos(Euler(1)) - Wb(3) * sin(Euler(1));
w3 = Wb(2) * sin(Euler(1)) / cos(Euler(2)) + Wb(3) * cos(Euler(1)) / cos(Euler(2));

Vel = [w1 w2 w3];

== matlab function Control_model_matching_no_lineal/Estimacion/IMU 3/Filtro pasa bajos  acelerometro/MATLAB Function1 ==
  settings: updateMethod=DISCRETE
  data: In input; Fc input; Out output; Ts input
function Out  = LowPassFilterP2(In, Fc, Ts)

persistent b0 b1 b2 a1 a2 a0 in1 in2 out1 out2

if isempty(b0)
    ohm     = 2 * pi * Fc;
    damping = 1 / (sqrt(2));

    b2 = Ts^2 * ohm^2;
    b1 = 2.0 * b2;
    b0 = b2;

    a2 = 4.0 + 4.0 * damping * ohm * Ts + b2;
    a1 = -8.0 + b1;
    a0 = 4.0 - 4.0 * damping * ohm * Ts + b2;

    in1  = 0;
    in2  = 0;
    out1 = 0;
    out2 = 0;
end

Out = (b2 * In + b1 * in1 + b0 * in2 - a1 * out1 - a0 * out2) / a2;

in2  = in1;
in1  = In;
out2 = out1;
out1 = Out;

== matlab function Control_model_matching_no_lineal/Estimacion/IMU 3/Filtro pasa bajos  acelerometro/MATLAB Function2 ==
  settings: updateMethod=DISCRETE
  data: In input; Fc input; Out output; Ts input
function Out  = LowPassFilterP2(In, Fc, Ts)

persistent b0 b1 b2 a1 a2 a0 in1 in2 out1 out2

if isempty(b0)
    ohm     = 2 * pi * Fc;
    damping = 1 / (sqrt(2));

    b2 = Ts^2 * ohm^2;
    b1 = 2.0 * b2;
    b0 = b2;

    a2 = 4.0 + 4.0 * damping * ohm * Ts + b2;
    a1 = -8.0 + b1;
    a0 = 4.0 - 4.0 * damping * ohm * Ts + b2;

    in1  = 0;
    in2  = 0;
    out1 = 0;
    out2 = 0;
end

Out = (b2 * In + b1 * in1 + b0 * in2 - a1 * out1 - a0 * out2) / a2;

in2  = in1;
in1  = In;
out2 = out1;
out1 = Out;

== matlab function Control_model_matching_no_lineal/Estimacion/IMU 3/Filtro pasa bajos  acelerometro/MATLAB Function3 ==
  settings: updateMethod=DISCRETE
  data: In input; Fc input; Out output; Ts input
function Out  = LowPassFilterP1(In, Fc, Ts)

persistent b0 b1 a0 a1 in1 out1

if isempty(b0)
    ohm = 2.0 * pi * Fc;

    b1 = ohm * Ts;
    b0 = b1;
    a1 = 2.0 + b1;
    a0 = b1 - 2.0;

    in1  = 0;
    out1 = 0;
end

Out = (b1 * In + b0 * in1 - a0 * out1) / a1;

in1  = In;
out1 = Out;

== matlab function Control_model_matching_no_lineal/Estimacion/IMU 3/Filtro pasa bajos  acelerometro/MATLAB Function4 ==
  settings: updateMethod=DISCRETE
  data: In input; Fc input; Out output; Ts input
function Out  = LowPassFilterP1(In, Fc, Ts)

persistent b0 b1 a0 a1 in1 out1

if isempty(b0)
    ohm = 2.0 * pi * Fc;

    b1 = ohm * Ts;
    b0 = b1;
    a1 = 2.0 + b1;
    a0 = b1 - 2.0;

    in1  = 0;
    out1 = 0;
end

Out = (b1 * In + b0 * in1 - a0 * out1) / a1;

in1  = In;
out1 = Out;

== matlab function Control_model_matching_no_lineal/Estimacion/IMU 3/Filtro pasa bajos  acelerometro/MATLAB Function5 ==
  settings: updateMethod=DISCRETE
  data: In input; Fc input; Out output; Ts input
function Out  = LowPassFilterP2(In, Fc, Ts)

persistent b0 b1 b2 a1 a2 a0 in1 in2 out1 out2

if isempty(b0)
    ohm     = 2 * pi * Fc;
    damping = 1 / (sqrt(2));

    b2 = Ts^2 * ohm^2;
    b1 = 2.0 * b2;
    b0 = b2;

    a2 = 4.0 + 4.0 * damping * ohm * Ts + b2;
    a1 = -8.0 + b1;
    a0 = 4.0 - 4.0 * damping * ohm * Ts + b2;

    in1  = 0;
    in2  = 0;
    out1 = 0;
    out2 = 0;
end

Out = (b2 * In + b1 * in1 + b0 * in2 - a1 * out1 - a0 * out2) / a2;

in2  = in1;
in1  = In;
out2 = out1;
out1 = Out;

== matlab function Control_model_matching_no_lineal/Estimacion/IMU 3/Filtro pasa bajos  acelerometro/MATLAB Function6 ==
  settings: updateMethod=DISCRETE
  data: In input; Fc input; Out output; Ts input
function Out  = LowPassFilterP1(In, Fc, Ts)

persistent b0 b1 a0 a1 in1 out1

if isempty(b0)
    ohm = 2.0 * pi * Fc;

    b1 = ohm * Ts;
    b0 = b1;
    a1 = 2.0 + b1;
    a0 = b1 - 2.0;

    in1  = 0;
    out1 = 0;
end

Out = (b1 * In + b0 * in1 - a0 * out1) / a1;

in1  = In;
out1 = Out;

== matlab function Control_model_matching_no_lineal/Estimacion/IMU 3/Filtro pasa bajos giroscopio/MATLAB Function1 ==
  settings: updateMethod=DISCRETE
  data: In input; Fc input; Out output; Ts input
function Out  = LowPassFilterP2(In, Fc, Ts)

persistent b0 b1 b2 a1 a2 a0 in1 in2 out1 out2

if isempty(b0)
    ohm     = 2 * pi * Fc;
    damping = 1 / (sqrt(2));

    b2 = Ts^2 * ohm^2;
    b1 = 2.0 * b2;
    b0 = b2;

    a2 = 4.0 + 4.0 * damping * ohm * Ts + b2;
    a1 = -8.0 + b1;
    a0 = 4.0 - 4.0 * damping * ohm * Ts + b2;

    in1  = 0;
    in2  = 0;
    out1 = 0;
    out2 = 0;
end

Out = (b2 * In + b1 * in1 + b0 * in2 - a1 * out1 - a0 * out2) / a2;

in2  = in1;
in1  = In;
out2 = out1;
out1 = Out;

== matlab function Control_model_matching_no_lineal/Estimacion/IMU 3/Filtro pasa bajos giroscopio/MATLAB Function2 ==
  settings: updateMethod=DISCRETE
  data: In input; Fc input; Out output; Ts input
function Out  = LowPassFilterP2(In, Fc, Ts)

persistent b0 b1 b2 a1 a2 a0 in1 in2 out1 out2

if isempty(b0)
    ohm     = 2 * pi * Fc;
    damping = 1 / (sqrt(2));

    b2 = Ts^2 * ohm^2;
    b1 = 2.0 * b2;
    b0 = b2;

    a2 = 4.0 + 4.0 * damping * ohm * Ts + b2;
    a1 = -8.0 + b1;
    a0 = 4.0 - 4.0 * damping * ohm * Ts + b2;

    in1  = 0;
    in2  = 0;
    out1 = 0;
    out2 = 0;
end

Out = (b2 * In + b1 * in1 + b0 * in2 - a1 * out1 - a0 * out2) / a2;

in2  = in1;
in1  = In;
out2 = out1;
out1 = Out;

== matlab function Control_model_matching_no_lineal/Estimacion/IMU 3/Filtro pasa bajos giroscopio/MATLAB Function3 ==
  settings: updateMethod=DISCRETE
  data: In input; Fc input; Out output; Ts input
function Out  = LowPassFilterP1(In, Fc, Ts)

persistent b0 b1 a0 a1 in1 out1

if isempty(b0)
    ohm = 2.0 * pi * Fc;

    b1 = ohm * Ts;
    b0 = b1;
    a1 = 2.0 + b1;
    a0 = b1 - 2.0;

    in1  = 0;
    out1 = 0;
end

Out = (b1 * In + b0 * in1 - a0 * out1) / a1;

in1  = In;
out1 = Out;

== matlab function Control_model_matching_no_lineal/Estimacion/IMU 3/Filtro pasa bajos giroscopio/MATLAB Function4 ==
  settings: updateMethod=DISCRETE
  data: In input; Fc input; Out output; Ts input
function Out  = LowPassFilterP1(In, Fc, Ts)

persistent b0 b1 a0 a1 in1 out1

if isempty(b0)
    ohm = 2.0 * pi * Fc;

    b1 = ohm * Ts;
    b0 = b1;
    a1 = 2.0 + b1;
    a0 = b1 - 2.0;

    in1  = 0;
    out1 = 0;
end

Out = (b1 * In + b0 * in1 - a0 * out1) / a1;

in1  = In;
out1 = Out;

== matlab function Control_model_matching_no_lineal/Sistema de control/PID pitch/MATLAB Function ==
  data: kp input; u output; ki input; kd input; kff input; limIntegral input; limTotal input; setPoint input; sensor input; sensorDerivada input; habIntegral input; tiempo input
function u = ControlPID(kp, ki, kd, kff, limIntegral, limTotal, setPoint, sensor, sensorDerivada, habIntegral, tiempo)

persistent integral tiempoAnterior

if isempty(integral)
    integral = 0;
    tiempoAnterior = 0;
end

dt = tiempo - tiempoAnterior;
tiempoAnterior = tiempo;

error  = setPoint - sensor;
salida = error * kp + ki - sensorDerivada * kd + setPoint * kff;

if habIntegral 
    integral = integral + error * dt * ki;

    if integral > limIntegral
        integral = limIntegral;
    elseif integral < -limIntegral
        integral = -limIntegral;
    end
end

if salida > limTotal
    salida = limTotal;
elseif salida < -limTotal
    salida = -limTotal;
end

u = salida;

== matlab function Control_model_matching_no_lineal/Sistema de control/PID roll/MATLAB Function ==
  data: kp input; u output; ki input; kd input; kff input; limIntegral input; limTotal input; setPoint input; sensor input; sensorDerivada input; habIntegral input; tiempo input
function u = ControlPID(kp, ki, kd, kff, limIntegral, limTotal, setPoint, sensor, sensorDerivada, habIntegral, tiempo)

persistent integral tiempoAnterior

if isempty(integral)
    integral = 0;
    tiempoAnterior = 0;
end

dt = tiempo - tiempoAnterior;
tiempoAnterior = tiempo;

error  = setPoint - sensor;
salida = error * kp + ki - sensorDerivada * kd + setPoint * kff;

if habIntegral 
    integral = integral + error * dt * ki;

    if integral > limIntegral
        integral = limIntegral;
    elseif integral < -limIntegral
        integral = -limIntegral;
    end
end

if salida > limTotal
    salida = limTotal;
elseif salida < -limTotal
    salida = -limTotal;
end

u = salida;

== matlab function Control_model_matching_no_lineal/Sistema de control/PID roll velocidad/MATLAB Function ==
  data: kp input; u output; ki input; kd input; kff input; limIntegral input; limTotal input; setpoint input; sensor input; sensorDerivada input; habIntegral input; tiempo input
function u = ControlPID(kp, ki, kd, kff, limIntegral, limTotal, setpoint, sensor, sensorDerivada, habIntegral, tiempo)

persistent integral tiempoAnterior

if isempty(integral)
    integral = 0;
    tiempoAnterior = 0;
end

dt = tiempo - tiempoAnterior;
tiempoAnterior = tiempo;

error  = setpoint - sensor;
salida = error * kp + ki - sensorDerivada * kd + setpoint * kff;

if habIntegral 
    integral = integral + error * dt * ki;

    if integral > limIntegral
        integral = limIntegral;
    elseif integral < -limIntegral
        integral = -limIntegral;
    end
end

if salida > limTotal
    salida = limTotal;
elseif salida < -limTotal
    salida = -limTotal;
end

u = salida;

== matlab function Control_model_matching_no_lineal/Sistema de control/PID pitch velocidad/MATLAB Function ==
  data: kp input; u output; ki input; kd input; kff input; limIntegral input; limTotal input; setPoint input; sensor input; sensorDerivada input; habIntegral input; tiempo input
function u = ControlPID(kp, ki, kd, kff, limIntegral, limTotal, setPoint, sensor, sensorDerivada, habIntegral, tiempo)

persistent integral tiempoAnterior

if isempty(integral)
    integral = 0;
    tiempoAnterior = 0;
end

dt = tiempo - tiempoAnterior;
tiempoAnterior = tiempo;

error  = setPoint - sensor;
salida = error * kp + ki - sensorDerivada * kd + setPoint * kff;

if habIntegral 
    integral = integral + error * dt * ki;

    if integral > limIntegral
        integral = limIntegral;
    elseif integral < -limIntegral
        integral = -limIntegral;
    end
end

if salida > limTotal
    salida = limTotal;
elseif salida < -limTotal
    salida = -limTotal;
end

u = salida;

== matlab function Control_model_matching_no_lineal/Sistema de control/PID yaw/MATLAB Function ==
  data: kp input; u output; ki input; kd input; kff input; limIntegral input; limTotal input; setPoint input; sensor input; sensorDerivada input; habIntegral input; tiempo input
function u = ControlPID(kp, ki, kd, kff, limIntegral, limTotal, setPoint, sensor, sensorDerivada, habIntegral, tiempo)

persistent integral tiempoAnterior

if isempty(integral)
    integral = 0;
    tiempoAnterior = 0;
end

dt = tiempo - tiempoAnterior;
tiempoAnterior = tiempo;

error  = setPoint - sensor;
salida = error * kp + ki - sensorDerivada * kd + setPoint * kff;

if habIntegral 
    integral = integral + error * dt * ki;

    if integral > limIntegral
        integral = limIntegral;
    elseif integral < -limIntegral
        integral = -limIntegral;
    end
end

if salida > limTotal
    salida = limTotal;
elseif salida < -limTotal
    salida = -limTotal;
end

u = salida;

== matlab function Control_model_matching_no_lineal/Sistema de control/PID yaw velocidad/MATLAB Function ==
  data: kp input; u output; ki input; kd input; kff input; limIntegral input; limTotal input; setPoint input; sensor input; sensorDerivada input; habIntegral input; tiempo input
function u = ControlPID(kp, ki, kd, kff, limIntegral, limTotal, setPoint, sensor, sensorDerivada, habIntegral, tiempo)

persistent integral tiempoAnterior

if isempty(integral)
    integral = 0;
    tiempoAnterior = 0;
end

dt = tiempo - tiempoAnterior;
tiempoAnterior = tiempo;

error  = setPoint - sensor;
salida = error * kp + ki - sensorDerivada * kd + setPoint * kff;

if habIntegral 
    integral = integral + error * dt * ki;

    if integral > limIntegral
        integral = limIntegral;
    elseif integral < -limIntegral
        integral = -limIntegral;
    end
end

if salida > limTotal
    salida = limTotal;
elseif salida < -limTotal
    salida = -limTotal;
end

u = salida;

== matlab function Control_model_matching_no_lineal/Sistema de control/MATLAB Function2 ==
  data: Euler input; Wb output; Vel input
function Wb = RotacionVelTB(Euler, Vel)

w = [0 0 0]';

w(1) = Vel(1) - sin(Euler(2)) * Vel(3);
w(2) = cos(Euler(1)) * Vel(2)   + sin(Euler(1)) * cos(Euler(2)) * Vel(3);
w(3) = - sin(Euler(1)) * Vel(2) + cos(Euler(2)) * cos(Euler(1)) * Vel(3);

Wb = w;

== matlab function Control_model_matching_no_lineal/Estimacion/IMU 3/Filtro pasa bajos giroscopio/MATLAB Function5 ==
  settings: updateMethod=DISCRETE
  data: In input; Fc input; Out output; Ts input
function Out  = LowPassFilterP2(In, Fc, Ts)

persistent b0 b1 b2 a1 a2 a0 in1 in2 out1 out2

if isempty(b0)
    ohm     = 2 * pi * Fc;
    damping = 1 / (sqrt(2));

    b2 = Ts^2 * ohm^2;
    b1 = 2.0 * b2;
    b0 = b2;

    a2 = 4.0 + 4.0 * damping * ohm * Ts + b2;
    a1 = -8.0 + b1;
    a0 = 4.0 - 4.0 * damping * ohm * Ts + b2;

    in1  = 0;
    in2  = 0;
    out1 = 0;
    out2 = 0;
end

Out = (b2 * In + b1 * in1 + b0 * in2 - a1 * out1 - a0 * out2) / a2;

in2  = in1;
in1  = In;
out2 = out1;
out1 = Out;

== matlab function Control_model_matching_no_lineal/Estimacion/IMU 1/Filtro pasa bajos  acelerometro/MATLAB Function2 ==
  settings: updateMethod=DISCRETE
  data: In input; Fc input; Out output; Ts input
function Out  = LowPassFilterP2(In, Fc, Ts)

persistent b0 b1 b2 a1 a2 a0 in1 in2 out1 out2

if isempty(b0)
    ohm     = 2 * pi * Fc;
    damping = 1 / (sqrt(2));

    b2 = Ts^2 * ohm^2;
    b1 = 2.0 * b2;
    b0 = b2;

    a2 = 4.0 + 4.0 * damping * ohm * Ts + b2;
    a1 = -8.0 + b1;
    a0 = 4.0 - 4.0 * damping * ohm * Ts + b2;

    in1  = 0;
    in2  = 0;
    out1 = 0;
    out2 = 0;
end

Out = (b2 * In + b1 * in1 + b0 * in2 - a1 * out1 - a0 * out2) / a2;

in2  = in1;
in1  = In;
out2 = out1;
out1 = Out;

== matlab function Control_model_matching_no_lineal/Estimacion/IMU 1/Filtro pasa bajos  acelerometro/MATLAB Function3 ==
  settings: updateMethod=DISCRETE
  data: In input; Fc input; Out output; Ts input
function Out  = LowPassFilterP1(In, Fc, Ts)

persistent b0 b1 a0 a1 in1 out1

if isempty(b0)
    ohm = 2.0 * pi * Fc;

    b1 = ohm * Ts;
    b0 = b1;
    a1 = 2.0 + b1;
    a0 = b1 - 2.0;

    in1  = 0;
    out1 = 0;
end

Out = (b1 * In + b0 * in1 - a0 * out1) / a1;

in1  = In;
out1 = Out;

== matlab function Control_model_matching_no_lineal/Estimacion/IMU 1/Filtro pasa bajos  acelerometro/MATLAB Function4 ==
  settings: updateMethod=DISCRETE
  data: In input; Fc input; Out output; Ts input
function Out  = LowPassFilterP1(In, Fc, Ts)

persistent b0 b1 a0 a1 in1 out1

if isempty(b0)
    ohm = 2.0 * pi * Fc;

    b1 = ohm * Ts;
    b0 = b1;
    a1 = 2.0 + b1;
    a0 = b1 - 2.0;

    in1  = 0;
    out1 = 0;
end

Out = (b1 * In + b0 * in1 - a0 * out1) / a1;

in1  = In;
out1 = Out;

== matlab function Control_model_matching_no_lineal/Estimacion/IMU 1/Filtro pasa bajos  acelerometro/MATLAB Function5 ==
  settings: updateMethod=DISCRETE
  data: In input; Fc input; Out output; Ts input
function Out  = LowPassFilterP2(In, Fc, Ts)

persistent b0 b1 b2 a1 a2 a0 in1 in2 out1 out2

if isempty(b0)
    ohm     = 2 * pi * Fc;
    damping = 1 / (sqrt(2));

    b2 = Ts^2 * ohm^2;
    b1 = 2.0 * b2;
    b0 = b2;

    a2 = 4.0 + 4.0 * damping * ohm * Ts + b2;
    a1 = -8.0 + b1;
    a0 = 4.0 - 4.0 * damping * ohm * Ts + b2;

    in1  = 0;
    in2  = 0;
    out1 = 0;
    out2 = 0;
end

Out = (b2 * In + b1 * in1 + b0 * in2 - a1 * out1 - a0 * out2) / a2;

in2  = in1;
in1  = In;
out2 = out1;
out1 = Out;

== matlab function Control_model_matching_no_lineal/Estimacion/IMU 1/Filtro pasa bajos  acelerometro/MATLAB Function6 ==
  settings: updateMethod=DISCRETE
  data: In input; Fc input; Out output; Ts input
function Out  = LowPassFilterP1(In, Fc, Ts)

persistent b0 b1 a0 a1 in1 out1

if isempty(b0)
    ohm = 2.0 * pi * Fc;

    b1 = ohm * Ts;
    b0 = b1;
    a1 = 2.0 + b1;
    a0 = b1 - 2.0;

    in1  = 0;
    out1 = 0;
end

Out = (b1 * In + b0 * in1 - a0 * out1) / a1;

in1  = In;
out1 = Out;

== matlab function Control_model_matching_no_lineal/Estimacion/Filtro pasa bajos acel angular/MATLAB Function1 ==
  settings: updateMethod=DISCRETE
  data: In input; Fc input; Out output; Ts input
function Out  = LowPassFilterP2(In, Fc, Ts)

persistent b0 b1 b2 a1 a2 a0 in1 in2 out1 out2

if isempty(b0)
    ohm     = 2 * pi * Fc;
    damping = 1 / (sqrt(2));

    b2 = Ts^2 * ohm^2;
    b1 = 2.0 * b2;
    b0 = b2;

    a2 = 4.0 + 4.0 * damping * ohm * Ts + b2;
    a1 = -8.0 + b1;
    a0 = 4.0 - 4.0 * damping * ohm * Ts + b2;

    in1  = 0;
    in2  = 0;
    out1 = 0;
    out2 = 0;
end

Out = (b2 * In + b1 * in1 + b0 * in2 - a1 * out1 - a0 * out2) / a2;

in2  = in1;
in1  = In;
out2 = out1;
out1 = Out;

== matlab function Control_model_matching_no_lineal/Estimacion/Filtro pasa bajos acel angular/MATLAB Function2 ==
  settings: updateMethod=DISCRETE
  data: In input; Fc input; Out output; Ts input
function Out  = LowPassFilterP2(In, Fc, Ts)

persistent b0 b1 b2 a1 a2 a0 in1 in2 out1 out2

if isempty(b0)
    ohm     = 2 * pi * Fc;
    damping = 1 / (sqrt(2));

    b2 = Ts^2 * ohm^2;
    b1 = 2.0 * b2;
    b0 = b2;

    a2 = 4.0 + 4.0 * damping * ohm * Ts + b2;
    a1 = -8.0 + b1;
    a0 = 4.0 - 4.0 * damping * ohm * Ts + b2;

    in1  = 0;
    in2  = 0;
    out1 = 0;
    out2 = 0;
end

Out = (b2 * In + b1 * in1 + b0 * in2 - a1 * out1 - a0 * out2) / a2;

in2  = in1;
in1  = In;
out2 = out1;
out1 = Out;

== matlab function Control_model_matching_no_lineal/Estimacion/Filtro pasa bajos acel angular/MATLAB Function3 ==
  settings: updateMethod=DISCRETE
  data: In input; Fc input; Out output; Ts input
function Out  = LowPassFilterP1(In, Fc, Ts)

persistent b0 b1 a0 a1 in1 out1

if isempty(b0)
    ohm = 2.0 * pi * Fc;

    b1 = ohm * Ts;
    b0 = b1;
    a1 = 2.0 + b1;
    a0 = b1 - 2.0;

    in1  = 0;
    out1 = 0;
end

Out = (b1 * In + b0 * in1 - a0 * out1) / a1;

in1  = In;
out1 = Out;

== matlab function Control_model_matching_no_lineal/Estimacion/Filtro pasa bajos acel angular/MATLAB Function4 ==
  settings: updateMethod=DISCRETE
  data: In input; Fc input; Out output; Ts input
function Out  = LowPassFilterP1(In, Fc, Ts)

persistent b0 b1 a0 a1 in1 out1

if isempty(b0)
    ohm = 2.0 * pi * Fc;

    b1 = ohm * Ts;
    b0 = b1;
    a1 = 2.0 + b1;
    a0 = b1 - 2.0;

    in1  = 0;
    out1 = 0;
end

Out = (b1 * In + b0 * in1 - a0 * out1) / a1;

in1  = In;
out1 = Out;

== matlab function Control_model_matching_no_lineal/Estimacion/Filtro pasa bajos acel angular/MATLAB Function5 ==
  settings: updateMethod=DISCRETE
  data: In input; Fc input; Out output; Ts input
function Out  = LowPassFilterP2(In, Fc, Ts)

persistent b0 b1 b2 a1 a2 a0 in1 in2 out1 out2

if isempty(b0)
    ohm     = 2 * pi * Fc;
    damping = 1 / (sqrt(2));

    b2 = Ts^2 * ohm^2;
    b1 = 2.0 * b2;
    b0 = b2;

    a2 = 4.0 + 4.0 * damping * ohm * Ts + b2;
    a1 = -8.0 + b1;
    a0 = 4.0 - 4.0 * damping * ohm * Ts + b2;

    in1  = 0;
    in2  = 0;
    out1 = 0;
    out2 = 0;
end

Out = (b2 * In + b1 * in1 + b0 * in2 - a1 * out1 - a0 * out2) / a2;

in2  = in1;
in1  = In;
out2 = out1;
out1 = Out;

== matlab function Control_model_matching_no_lineal/Estimacion/Filtro pasa bajos acel angular/MATLAB Function6 ==
  settings: updateMethod=DISCRETE
  data: In input; Fc input; Out output; Ts input
function Out  = LowPassFilterP1(In, Fc, Ts)

persistent b0 b1 a0 a1 in1 out1

if isempty(b0)
    ohm = 2.0 * pi * Fc;

    b1 = ohm * Ts;
    b0 = b1;
    a1 = 2.0 + b1;
    a0 = b1 - 2.0;

    in1  = 0;
    out1 = 0;
end

Out = (b1 * In + b0 * in1 - a0 * out1) / a1;

in1  = In;
out1 = Out;
